simulink model "CRITIS_1_full"  (R2022b)
settings: Solver=VariableStepAuto  StartTime=0.0  StopTime=7  RelTol=1e-3
(part 8 of 13)

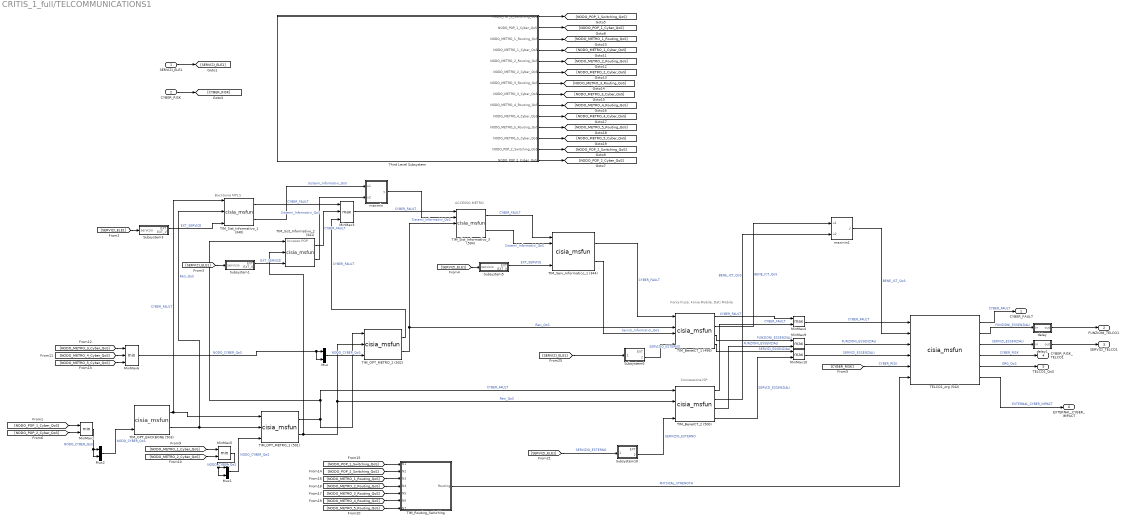
== system CRITIS_1_full/TELCOMMUNICATIONS1 ==
  note: Fonia Fissa, Fonia Mobile, Dati Mobile
  note: Connessione ISP
  note: Backbone MPLS
  note: Accesso POP
  note: ACCESSO METRO
  SERVIZI_ELE1 : Inport
  CYBER_RISK : Inport  Port=2
  MinMax1 : MinMax  Inputs=2
  MinMax10 : MinMax  Function=max  Inputs=2
  MinMax3 : MinMax  Function=max  Inputs=3
  MinMax4 : MinMax  Function=max  Inputs=2
  MinMax5 : MinMax  Inputs=2
  MinMax6 : MinMax  Inputs=3
  MinMax9 : MinMax  Function=max  Inputs=2
  Mux : Mux  Inputs=2
  Mux1 : Mux  Inputs=2
  Mux2 : Mux  Inputs=2
  Subsystem1 : Subsystem  mask{num_serv=1, operation1=All services required, operation2=All providers required, out_service=none, consumed1=[1 0 0 0 0 0 0 0 0 0]}
      mask prompts: num_serv "Providers in input"; operation1 "For each single service provider"; operation2 "Among providers"; out_service "Vectorial output"; consumed1 "Required 1"
      mask TypeOptions num_serv: 1
      mask TypeOptions operation1: All services required | At least one
      mask TypeOptions operation2: All providers required
      mask TypeOptions out_service: none | S1 | S2 | S3 | S4 | S5 | S6 | S7 | S8 | S9 | S10 | F1 | F2 | F3 | F4 | F5 | F6 | F7 | F8 | F9 | F10
  Subsystem10 : Subsystem  mask{num_serv=1, operation1=All services required, operation2=All providers required, out_service=S4, consumed1=[1 0 0 0 0 0 0 0 0 0]}
      mask prompts: num_serv "Providers in input"; operation1 "For each single service provider"; operation2 "Among providers"; out_service "Vectorial output"; consumed1 "Required 1"
      mask TypeOptions num_serv: 1
      mask TypeOptions operation1: All services required | At least one
      mask TypeOptions operation2: All providers required
      mask TypeOptions out_service: none | S1 | S2 | S3 | S4 | S5 | S6 | S7 | S8 | S9 | S10 | F1 | F2 | F3 | F4 | F5 | F6 | F7 | F8 | F9 | F10
  Subsystem3 : Subsystem  mask{num_serv=1, operation1=All services required, operation2=All providers required, out_service=none, consumed1=[1 0 0 0 0 0 0 0 0 0]}
      mask prompts: num_serv "Providers in input"; operation1 "For each single service provider"; operation2 "Among providers"; out_service "Vectorial output"; consumed1 "Required 1"
      mask TypeOptions num_serv: 1
      mask TypeOptions operation1: All services required | At least one
      mask TypeOptions operation2: All providers required
      mask TypeOptions out_service: none | S1 | S2 | S3 | S4 | S5 | S6 | S7 | S8 | S9 | S10 | F1 | F2 | F3 | F4 | F5 | F6 | F7 | F8 | F9 | F10
  Subsystem5 : Subsystem  mask{num_serv=1, operation1=All services required, operation2=All providers required, out_service=none, consumed1=[1 0 0 0 0 0 0 0 0 0]}
      mask prompts: num_serv "Providers in input"; operation1 "For each single service provider"; operation2 "Among providers"; out_service "Vectorial output"; consumed1 "Required 1"
      mask TypeOptions num_serv: 1
      mask TypeOptions operation1: All services required | At least one
      mask TypeOptions operation2: All providers required
      mask TypeOptions out_service: none | S1 | S2 | S3 | S4 | S5 | S6 | S7 | S8 | S9 | S10 | F1 | F2 | F3 | F4 | F5 | F6 | F7 | F8 | F9 | F10
  Subsystem6 : Subsystem  mask{num_serv=1, operation1=All services required, operation2=All providers required, out_service=S1, consumed1=[1 0 0 0 0 0 0 0 0 0]}
      mask prompts: num_serv "Providers in input"; operation1 "For each single service provider"; operation2 "Among providers"; out_service "Vectorial output"; consumed1 "Required 1"
      mask TypeOptions num_serv: 1
      mask TypeOptions operation1: All services required | At least one
      mask TypeOptions operation2: All providers required
      mask TypeOptions out_service: none | S1 | S2 | S3 | S4 | S5 | S6 | S7 | S8 | S9 | S10 | F1 | F2 | F3 | F4 | F5 | F6 | F7 | F8 | F9 | F10
  TELCO1_org (542) : M-S-Function  FunctionName=cisia_msfun  Parameters=Parameter1, Parameter2, Parameter3, resources, Parameter10, codeupdate, step_received, step_computed, dynamic_computed, step_sended, id_entity, id_project, id_type, name_type, color  mask(S-function:msfcn_unit_delay){Parameter1='TELCO1_org', Parameter2=1, Parameter3='Iside', resources=|, Parameter10=off, codeupdate=off, step_received=|, step_computed=, dynamic_computed=, step_sended=|, id_entity=542, id_project=14, id_type=118, name_type=Organization, color=#A2142F}
      mask resources=|
      | *** INPUT RESOURCES ***
      | NUM_INPUTS 6
      | CYBER_FAULT (25)
      | BENE_ICT_QoS (2)
      | FUNZIONI_ESSENZIALI (10)
      | SERVIZI_ESSENZIALI (10)
      | CYBER_RISK (3)
      | PHYSICAL_STRENGTH (1)
      |
      | *** STATE VARIABLES ***
      | NUM_VARIABLES 35
      | Operative_Level(NUMERIC)(1)(1)
      | Dos_attack(NUMERIC)(1)(0)
      | MITM_attack(NUMERIC)(1)(0)
      | Virus_Attack(NUMERIC)(1)(0)
      | Port_Scan_Attack(NUMERIC)(1)(0)
      | Cyber_Fault(NUMERIC_ARRAY)(25)(0  0  0  0  0  0  0  0  0  0  0  0  0  0  0  0  0  0  0  0  0  0  0  0  0)
      | BGP_hijacking(NUMERIC)(1)(0)
      | Mechanical_Fault(NUMERIC)(1)(0)
      | Unauthorized_Access(NUMERIC)(1)(0)
      | Conn_Fault(NUMERIC)(1)(0)
      | BotNet_Attack(NUMERIC)(1)(0)
      | Data_Corruption(NUMERIC)(1)(0)
      | Rouge_Access(NUMERIC)(1)(0)
      | syslog_adm_login(NUMERIC)(1)(0)
      | SW_Change(NUMERIC)(1)(0)
      | Config_Change(NUMERIC)(1)(0)
      | Port_Saturation(NUMERIC)(1)(0)
      | Congestion_Fault(NUMERIC)(1)(0)
      | Physical_Fault(NUMERIC)(1)(0)
      | Route_Poisoning(NUMERIC)(1)(0)
      | Interface_Down(NUMERIC)(1)(0)
      | Port_Isolation(NUMERIC)(1)(0)
      | Unknown_Device(NUMERIC)(1)(0)
      | USB_Device_Insertion(NUMERIC)(1)(0)
      | SW_Fault(NUMERIC)(1)(0)
      | Servizi_Essenziali(NUMERIC_ARRAY)(10)(0  0  0  0  0  0  0  0  0  0)
      | Funzioni_Essenziali(NUMERIC_ARRAY)(10)(0  0  0  0  0  0  0  0  0  0)
      | Internal_Cyber_Risk(NUMERIC)(1)(0)
      | Data_Breach(NUMERIC)(1)(0)
      | availability_fault(NUMERIC)(1)(0)
      | Ransomware(NUMERIC)(1)(0)
      | ExternalCyberFault(NUMERIC_ARRAY)(3)(0  0  0)
      | Op_Level2(NUMERIC_ARRAY)(2)(1  1)
      | Possibility_Value(NUMERIC)(1)(0)
      | Necessity_Value(NUMERIC)(1)(0)
      |
      | *** OUTPUT RESOURCES ***
      | NUM_OUTPUTS 6
      | CYBER_FAULT (25)
      | FUNZIONI_ESSENZIALI (10)
      | SERVIZI_ESSENZIALI (10)
      | CYBER_RISK (3)
      | ORG_QoS (2)
      | EXTERNAL_CYBER_IMPACT (1)
      mask step_received=|
      | cyber_event=zeros(1,25);
      | cyber_event(1)=Dos_attack;
      | cyber_event(2)=MITM_attack;
      | cyber_event(3)=Virus_Attack;
      | cyber_event(4)=Port_Scan_Attack;
      | cyber_event(5)=BGP_hijacking;
      | cyber_event(6)=BotNet_Attack;
      | cyber_event(7)=Data_Corruption;
      | cyber_event(8)=SW_Change;
      | cyber_event(9)=Config_Change;
      | cyber_event(10)=Port_Saturation;
      | cyber_event(11)=Data_Breach;
      | cyber_event(12)=Unauthorized_Access;
      | cyber_event(13)=Unknown_Device;
      | cyber_event(14)=Congestion_Fault;
      | cyber_event(15)=Interface_Down;
      | cyber_event(16)=Port_Isolation;
      | cyber_event(17)=Rouge_Access;
      | cyber_event(18)=Route_Poisoning;
      | cyber_event(19)=SW_Fault;
      | cyber_event(20)=syslog_adm_login;
      | cyber_event(21)=USB_Device_Insertion;
      | cyber_event(22)=Ransomware;
      | cyber_event(23)=0;
      | cyber_event(24)=0;
      | cyber_event(25)=0;
      |
      | Cyber_Fault=max(CYBER_FAULT, transpose(cyber_event));
      |
      |
      | Conn_Fault=max([Dos_attack BGP_hijacking Route_Poisoning Interface_Down Mechanical_Fault] );
      |
      |
      | Servizi_Essenziali=SERVIZI_ESSENZIALI;
      | Funzioni_Essenziali=FUNZIONI_ESSENZIALI;
      |
      | ExternalCyberFault=CYBER_RISK;
      |
      | Operative_Level=min([1-0.5*max(Cyber_Fault) mean(BENE_ICT_QoS) PHYSICAL_STRENGTH]);
      |
      |
      | Physical_Fault=1-PHYSICAL_STRENGTH;
      |
      | % Il primo elemento rappersenta possibility e si combima
      | % con il max in quanto rende conto del caso migliore
      | % (perche OL)
      |
      | Op_Level2(1)=  min([1-0.3*max(Cyber_Fault) BENE_ICT_QoS(1) PHYSICAL_STRENGTH]);
      |
      | % Il secondo elemento rappersenta necessity e si combima
      | % con il min in quanto rende conto del caso peggiore
      | % (perche OL)
      |
      | Op_Level2(2)= min([1-0.6*max(Cyber_Fault) BENE_ICT_QoS(2) PHYSICAL_STRENGTH]);
      |
      | Possibility_Value = Op_Level2(1);
      | Necessity_Value = Op_Level2(2);
      mask step_sended=|
      | SERVIZI_ESSENZIALI=Servizi_Essenziali*(1-Physical_Fault);
      | FUNZIONI_ESSENZIALI=Funzioni_Essenziali*(1-Physical_Fault);
      |
      |
      | ORG_QoS = Op_Level2;
      |
      | % Need to evaluate C-I-A from Cyber_Fault
      | integrity_fault=max([Cyber_Fault(7)  Cyber_Fault(8) Cyber_Fault(22)]);
      |
      | confidentiality_fault=max([Cyber_Fault(2)  Cyber_Fault(3)  Cyber_Fault(6)  Cyber_Fault(9) Cyber_Fault(22)]);
      |
      | availability_fault=max(Cyber_Fault);
      |
      |
      | % C-I-A
      | CYBER_RISK(1)=confidentiality_fault;
      | CYBER_RISK(2)=integrity_fault;
      | CYBER_RISK(3)=availability_fault;
      |
      | % Need to filter the propagable ones
      | CYBER_FAULT = Cyber_Fault;
      |
      |
      | % Need to map from external risks to internal ones
      | EXTERNAL_CYBER_IMPACT=max(ExternalCyberFault);
      mask prompts: Parameter1 "entity name"; Parameter2 "sampling time"; Parameter3 "project"; resources "input resources and state variables"; Parameter10 "Bring state variables to output"; codeupdate "update code from mask"
      mask help: This is a level-2 MATLAB file S-function which demonstrates CISIA entity
      mask DialogControl Container1 Prompt: All parameters
      mask Display: disp('Organization')
  TIM_BeneICT_1 (499) : M-S-Function  FunctionName=cisia_msfun  Parameters=Parameter1, Parameter2, Parameter3, resources, Parameter10, codeupdate, step_received, step_computed, dynamic_computed, step_sended, id_entity, id_project, id_type, name_type, color  mask(S-function:msfcn_unit_delay){Parameter1='TIM_BeneICT_1', Parameter2=1, Parameter3='Iside', resources=|, Parameter10=off, codeupdate=off, step_received=|, step_computed=, dynamic_computed=, step_sended=|, id_entity=499, id_project=14, id_type=108, name_type=BeneICT, color=#64D413}
      mask resources=|
      | *** INPUT RESOURCES ***
      | NUM_INPUTS 6
      | CYBER_FAULT (25)
      | Sistemi_Informativi_QoS (2)
      | Reti_QoS (2)
      | Servizi_Informatici_QoS (2)
      | BENE_ICT_QoS (2)
      | SERVIZIO_ESTERNO (20)
      |
      | *** STATE VARIABLES ***
      | NUM_VARIABLES 34
      | Operative_Level(NUMERIC)(1)(1)
      | Dos_attack(NUMERIC)(1)(0)
      | MITM_attack(NUMERIC)(1)(0)
      | Virus_Attack(NUMERIC)(1)(0)
      | Port_Scan_Attack(NUMERIC)(1)(0)
      | Cyber_Fault(NUMERIC_ARRAY)(25)(0  0  0  0  0  0  0  0  0  0  0  0  0  0  0  0  0  0  0  0  0  0  0  0  0)
      | BGP_hijacking(NUMERIC)(1)(0)
      | Unauthorized_Access(NUMERIC)(1)(0)
      | Consumed_Services(NUMERIC_ARRAY)(10)(0  0  0  0  0  0  0  0  0  0)
      | Service_Fault(NUMERIC)(1)(0)
      | BotNet_Attack(NUMERIC)(1)(0)
      | Data_Corruption(NUMERIC)(1)(0)
      | Rouge_Access(NUMERIC)(1)(0)
      | syslog_adm_login(NUMERIC)(1)(0)
      | SW_Change(NUMERIC)(1)(0)
      | Config_Change(NUMERIC)(1)(0)
      | Port_Saturation(NUMERIC)(1)(0)
      | Congestion_Fault(NUMERIC)(1)(0)
      | Route_Poisoning(NUMERIC)(1)(0)
      | Interface_Down(NUMERIC)(1)(0)
      | Port_Isolation(NUMERIC)(1)(0)
      | Unknown_Device(NUMERIC)(1)(0)
      | USB_Device_Insertion(NUMERIC)(1)(0)
      | SW_Fault(NUMERIC)(1)(0)
      | Servizi_Essenziali(NUMERIC_ARRAY)(10)(1  0  0  0  0  0  0  0  0  0)
      | Funzioni_Essenziali(NUMERIC_ARRAY)(10)(1  0  0  0  0  0  0  0  0  0)
      | Consumed_Functions(NUMERIC_ARRAY)(10)(0  0  0  0  0  0  0  0  0  0)
      | Internal_Cyber_Risk(NUMERIC)(1)(0)
      | Data_Breach(NUMERIC)(1)(0)
      | availability_fault(NUMERIC)(1)(0)
      | Ransomware(NUMERIC)(1)(0)
      | Op_Level2(NUMERIC_ARRAY)(2)(0  0)
      | Possibility_Value(NUMERIC)(1)(0)
      | Necessity_Value(NUMERIC)(1)(0)
      |
      | *** OUTPUT RESOURCES ***
      | NUM_OUTPUTS 4
      | CYBER_FAULT (25)
      | BENE_ICT_QoS (2)
      | FUNZIONI_ESSENZIALI (10)
      | SERVIZI_ESSENZIALI (10)
      mask step_received=|
      | cyber_event=zeros(1,25);
      | cyber_event(1)=Dos_attack;
      | cyber_event(2)=MITM_attack;
      | cyber_event(3)=Virus_Attack;
      | cyber_event(4)=Port_Scan_Attack;
      | cyber_event(5)=BGP_hijacking;
      | cyber_event(6)=BotNet_Attack;
      | cyber_event(7)=Data_Corruption;
      | cyber_event(8)=SW_Change;
      | cyber_event(9)=Config_Change;
      | cyber_event(10)=Port_Saturation;
      | cyber_event(11)=Data_Breach;
      | cyber_event(12)=Unauthorized_Access;
      | cyber_event(13)=Unknown_Device;
      | cyber_event(14)=Congestion_Fault;
      | cyber_event(15)=Interface_Down;
      | cyber_event(16)=Port_Isolation;
      | cyber_event(17)=Rouge_Access;
      | cyber_event(18)=Route_Poisoning;
      | cyber_event(19)=SW_Fault;
      | cyber_event(20)=syslog_adm_login;
      | cyber_event(21)=USB_Device_Insertion;
      | cyber_event(22)=Ransomware;
      | cyber_event(23)=0;
      | cyber_event(24)=0;
      | cyber_event(25)=0;
      |
      | Cyber_Fault=max(CYBER_FAULT, transpose(cyber_event));
      |
      | Consumed_Services=SERVIZIO_ESTERNO(1:10);
      | Consumed_Functions=SERVIZIO_ESTERNO(11:20);
      |
      | Service_Fault=max(abs(Servizi_Essenziali-Consumed_Services));
      |
      | availability_fault=1-min([(1-0.5*max(Cyber_Fault)) min(Reti_QoS) min(Sistemi_Informativi_QoS) min(Servizi_Informatici_QoS) min(BENE_ICT_QoS)]);
      |
      | Operative_Level=min([(1-0.5*max(Cyber_Fault)) mean(Reti_QoS) mean(Sistemi_Informativi_QoS) mean(Servizi_Informatici_QoS) mean(BENE_ICT_QoS) 1-Service_Fault]);
      |
      | % Il primo elemento rappersenta possibility e si combima
      | % con il max in quanto rende conto del caso migliore
      | % (perche OL)
      |
      | BNICT=BENE_ICT_QoS;
      |
      | Op_Level2(1)=  min([1-0.3*max(Cyber_Fault) max([use_elem(Reti_QoS,1) use_elem(Sistemi_Informativi_QoS,1) use_elem(Servizi_Informatici_QoS,1) use_elem(BENE_ICT_QoS,1)]) 1-Service_Fault]);
      |
      | % Il secondo elemento rappresenta necessity e si combima
      | % con il min in quanto rende conto del caso peggiore
      | % (perche OL)
      |
      |
      |
      | Op_Level2(2)= min([1-0.6*max(Cyber_Fault) min([use_elem(Reti_QoS,2) use_elem(Sistemi_Informativi_QoS,2) use_elem(Servizi_Informatici_QoS,2) use_elem(BENE_ICT_QoS,2)]) 1-Service_Fault]);
      |
      | Possibility_Value = Op_Level2(1);
      | Necessity_Value = Op_Level2(2);
      mask step_sended=|
      | CYBER_FAULT=Cyber_Fault;
      |
      | FUNZIONI_ESSENZIALI=(1-availability_fault)*Funzioni_Essenziali.*Consumed_Functions;
      |
      | SERVIZI_ESSENZIALI=(1-availability_fault)*Servizi_Essenziali.*Consumed_Services;
      |
      | BENE_ICT_QoS=Op_Level2;
      mask prompts: Parameter1 "entity name"; Parameter2 "sampling time"; Parameter3 "project"; resources "input resources and state variables"; Parameter10 "Bring state variables to output"; codeupdate "update code from mask"
      mask help: This is a level-2 MATLAB file S-function which demonstrates CISIA entity
      mask DialogControl Container1 Prompt: All parameters
      mask Display: disp('BeneICT');port_label('input',2,'\color{yellow}\spadesuit','texmode','on');port_label('input',5,'\color{yellow}\spadesuit','texmode','on')
  TIM_BeneICT_2 (500) : M-S-Function  FunctionName=cisia_msfun  Parameters=Parameter1, Parameter2, Parameter3, resources, Parameter10, codeupdate, step_received, step_computed, dynamic_computed, step_sended, id_entity, id_project, id_type, name_type, color  mask(S-function:msfcn_unit_delay){Parameter1='TIM_BeneICT_2', Parameter2=1, Parameter3='Iside', resources=|, Parameter10=off, codeupdate=off, step_received=|, step_computed=, dynamic_computed=, step_sended=|, id_entity=500, id_project=14, id_type=108, name_type=BeneICT, color=#64D413}
      mask resources=|
      | *** INPUT RESOURCES ***
      | NUM_INPUTS 6
      | CYBER_FAULT (25)
      | Sistemi_Informativi_QoS (2)
      | Reti_QoS (2)
      | Servizi_Informatici_QoS (2)
      | BENE_ICT_QoS (2)
      | SERVIZIO_ESTERNO (20)
      |
      | *** STATE VARIABLES ***
      | NUM_VARIABLES 34
      | Operative_Level(NUMERIC)(1)(1)
      | Dos_attack(NUMERIC)(1)(0)
      | MITM_attack(NUMERIC)(1)(0)
      | Virus_Attack(NUMERIC)(1)(0)
      | Port_Scan_Attack(NUMERIC)(1)(0)
      | Cyber_Fault(NUMERIC_ARRAY)(25)(0  0  0  0  0  0  0  0  0  0  0  0  0  0  0  0  0  0  0  0  0  0  0  0  0)
      | BGP_hijacking(NUMERIC)(1)(0)
      | Unauthorized_Access(NUMERIC)(1)(0)
      | Consumed_Services(NUMERIC_ARRAY)(10)(0  0  0  0  0  0  0  0  0  0)
      | Service_Fault(NUMERIC)(1)(0)
      | BotNet_Attack(NUMERIC)(1)(0)
      | Data_Corruption(NUMERIC)(1)(0)
      | Rouge_Access(NUMERIC)(1)(0)
      | syslog_adm_login(NUMERIC)(1)(0)
      | SW_Change(NUMERIC)(1)(0)
      | Config_Change(NUMERIC)(1)(0)
      | Port_Saturation(NUMERIC)(1)(0)
      | Congestion_Fault(NUMERIC)(1)(0)
      | Route_Poisoning(NUMERIC)(1)(0)
      | Interface_Down(NUMERIC)(1)(0)
      | Port_Isolation(NUMERIC)(1)(0)
      | Unknown_Device(NUMERIC)(1)(0)
      | USB_Device_Insertion(NUMERIC)(1)(0)
      | SW_Fault(NUMERIC)(1)(0)
      | Servizi_Essenziali(NUMERIC_ARRAY)(10)(0  0  0  1  0  0  0  0  0  0)
      | Funzioni_Essenziali(NUMERIC_ARRAY)(10)(1  0  0  0  0  0  0  0  0  0)
      | Consumed_Functions(NUMERIC_ARRAY)(10)(0  0  0  0  0  0  0  0  0  0)
      | Internal_Cyber_Risk(NUMERIC)(1)(0)
      | Data_Breach(NUMERIC)(1)(0)
      | availability_fault(NUMERIC)(1)(0)
      | Ransomware(NUMERIC)(1)(0)
      | Op_Level2(NUMERIC_ARRAY)(2)(0  0)
      | Possibility_Value(NUMERIC)(1)(0)
      | Necessity_Value(NUMERIC)(1)(0)
      |
      | *** OUTPUT RESOURCES ***
      | NUM_OUTPUTS 4
      | CYBER_FAULT (25)
      | BENE_ICT_QoS (2)
      | FUNZIONI_ESSENZIALI (10)
      | SERVIZI_ESSENZIALI (10)
      mask step_received=|
      | cyber_event=zeros(1,25);
      | cyber_event(1)=Dos_attack;
      | cyber_event(2)=MITM_attack;
      | cyber_event(3)=Virus_Attack;
      | cyber_event(4)=Port_Scan_Attack;
      | cyber_event(5)=BGP_hijacking;
      | cyber_event(6)=BotNet_Attack;
      | cyber_event(7)=Data_Corruption;
      | cyber_event(8)=SW_Change;
      | cyber_event(9)=Config_Change;
      | cyber_event(10)=Port_Saturation;
      | cyber_event(11)=Data_Breach;
      | cyber_event(12)=Unauthorized_Access;
      | cyber_event(13)=Unknown_Device;
      | cyber_event(14)=Congestion_Fault;
      | cyber_event(15)=Interface_Down;
      | cyber_event(16)=Port_Isolation;
      | cyber_event(17)=Rouge_Access;
      | cyber_event(18)=Route_Poisoning;
      | cyber_event(19)=SW_Fault;
      | cyber_event(20)=syslog_adm_login;
      | cyber_event(21)=USB_Device_Insertion;
      | cyber_event(22)=Ransomware;
      | cyber_event(23)=0;
      | cyber_event(24)=0;
      | cyber_event(25)=0;
      |
      | Cyber_Fault=max(CYBER_FAULT, transpose(cyber_event));
      |
      | Consumed_Services=SERVIZIO_ESTERNO(1:10);
      | Consumed_Functions=SERVIZIO_ESTERNO(11:20);
      |
      | Service_Fault=max(abs(Servizi_Essenziali-Consumed_Services));
      |
      | availability_fault=1-min([(1-0.5*max(Cyber_Fault)) min(Reti_QoS) min(Sistemi_Informativi_QoS) min(Servizi_Informatici_QoS) min(BENE_ICT_QoS)]);
      |
      | Operative_Level=min([(1-0.5*max(Cyber_Fault)) mean(Reti_QoS) mean(Sistemi_Informativi_QoS) mean(Servizi_Informatici_QoS) mean(BENE_ICT_QoS) 1-Service_Fault]);
      |
      | % Il primo elemento rappersenta possibility e si combima
      | % con il max in quanto rende conto del caso migliore
      | % (perche OL)
      |
      | BNICT=BENE_ICT_QoS;
      |
      | Op_Level2(1)=  min([1-0.3*max(Cyber_Fault) max([use_elem(Reti_QoS,1) use_elem(Sistemi_Informativi_QoS,1) use_elem(Servizi_Informatici_QoS,1) use_elem(BENE_ICT_QoS,1)]) 1-Service_Fault]);
      |
      | % Il secondo elemento rappresenta necessity e si combima
      | % con il min in quanto rende conto del caso peggiore
      | % (perche OL)
      |
      |
      |
      | Op_Level2(2)= min([1-0.6*max(Cyber_Fault) min([use_elem(Reti_QoS,2) use_elem(Sistemi_Informativi_QoS,2) use_elem(Servizi_Informatici_QoS,2) use_elem(BENE_ICT_QoS,2)]) 1-Service_Fault]);
      |
      | Possibility_Value = Op_Level2(1);
      | Necessity_Value = Op_Level2(2);
      mask step_sended=|
      | CYBER_FAULT=Cyber_Fault;
      |
      | FUNZIONI_ESSENZIALI=(1-availability_fault)*Funzioni_Essenziali.*Consumed_Functions;
      |
      | SERVIZI_ESSENZIALI=(1-availability_fault)*Servizi_Essenziali.*Consumed_Services;
      |
      | BENE_ICT_QoS=Op_Level2;
      mask prompts: Parameter1 "entity name"; Parameter2 "sampling time"; Parameter3 "project"; resources "input resources and state variables"; Parameter10 "Bring state variables to output"; codeupdate "update code from mask"
      mask help: This is a level-2 MATLAB file S-function which demonstrates CISIA entity
      mask DialogControl Container1 Prompt: All parameters
      mask Display: disp('BeneICT');port_label('input',2,'\color{yellow}\spadesuit','texmode','on');port_label('input',4,'\color{yellow}\spadesuit','texmode','on');port_label('input',5,'\color{yellow}\spadesuit','texmode','on')
  TIM_OPT_BACKBONE (503) : M-S-Function  FunctionName=cisia_msfun  Parameters=Parameter1, Parameter2, Parameter3, resources, Parameter10, codeupdate, step_received, step_computed, dynamic_computed, step_sended, id_entity, id_project, id_type, name_type, color  mask(S-function:msfcn_unit_delay){Parameter1='TIM_OPT_BACKBONE', Parameter2=1, Parameter3='Iside', resources=|, Parameter10=off, codeupdate=off, step_received=|, step_computed=, dynamic_computed=, step_sended=|, id_entity=503, id_project=14, id_type=82, name_type=Reti_Sito, color=#45B5ED}
      mask resources=|
      | *** INPUT RESOURCES ***
      | NUM_INPUTS 3
      | CYBER_FAULT (25)
      | Reti_QoS (2)
      | NODO_CYBER_QoS (2)
      |
      | *** STATE VARIABLES ***
      | NUM_VARIABLES 34
      | Operative_Level(NUMERIC)(1)(1)
      | Dos_attack(NUMERIC)(1)(0)
      | MITM_attack(NUMERIC)(1)(0)
      | Virus_Attack(NUMERIC)(1)(0)
      | Port_Scan_Attack(NUMERIC)(1)(0)
      | Cyber_Fault(NUMERIC_ARRAY)(25)(0  0  0  0  0  0  0  0  0  0  0  0  0  0  0  0  0  0  0  0  0  0  0  0  0)
      | BGP_hijacking(NUMERIC)(1)(0)
      | Mechanical_Fault(NUMERIC)(1)(0)
      | Unauthorized_Access(NUMERIC)(1)(0)
      | Conn_Fault(NUMERIC)(1)(0)
      | BotNet_Attack(NUMERIC)(1)(0)
      | Data_Corruption(NUMERIC)(1)(0)
      | Rouge_Access(NUMERIC)(1)(0)
      | syslog_adm_login(NUMERIC)(1)(0)
      | SW_Change(NUMERIC)(1)(0)
      | Config_Change(NUMERIC)(1)(0)
      | Port_Saturation(NUMERIC)(1)(0)
      | Congestion_Fault(NUMERIC)(1)(0)
      | Physical_Fault(NUMERIC)(1)(0)
      | Route2(NUMERIC)(1)(0)
      | Route_Poisoning(NUMERIC)(1)(0)
      | Interface_Down(NUMERIC)(1)(0)
      | Port_Isolation(NUMERIC)(1)(0)
      | Unknown_Device(NUMERIC)(1)(0)
      | USB_Device_Insertion(NUMERIC)(1)(0)
      | Risorsa(NUMERIC)(1)(0)
      | GEO_localization(STRING)(100)()
      | SW_Fault(NUMERIC)(1)(0)
      | Internal_Cyber_Risk(NUMERIC)(1)(0)
      | Data_Breach(NUMERIC)(1)(0)
      | Ransomware(NUMERIC)(1)(0)
      | Op_Level2(NUMERIC_ARRAY)(2)(0  0)
      | Possibility_Value(NUMERIC)(1)(0)
      | Necessity_Value(NUMERIC)(1)(0)
      |
      | *** OUTPUT RESOURCES ***
      | NUM_OUTPUTS 2
      | CYBER_FAULT (25)
      | Reti_QoS (2)
      mask step_received=|
      | cyber_event=zeros(1,25);
      | cyber_event(1)=Dos_attack;
      | cyber_event(2)=MITM_attack;
      | cyber_event(3)=Virus_Attack;
      | cyber_event(4)=Port_Scan_Attack;
      | cyber_event(5)=BGP_hijacking;
      | cyber_event(6)=BotNet_Attack;
      | cyber_event(7)=Data_Corruption;
      | cyber_event(8)=SW_Change;
      | cyber_event(9)=Config_Change;
      | cyber_event(10)=Port_Saturation;
      | cyber_event(11)=Data_Breach;
      | cyber_event(12)=Unauthorized_Access;
      | cyber_event(13)=Unknown_Device;
      | cyber_event(14)=Congestion_Fault;
      | cyber_event(15)=Interface_Down;
      | cyber_event(16)=Port_Isolation;
      | cyber_event(17)=Rouge_Access;
      | cyber_event(18)=Route_Poisoning;
      | cyber_event(19)=SW_Fault;
      | cyber_event(20)=syslog_adm_login;
      | cyber_event(21)=USB_Device_Insertion;
      | cyber_event(22)=Ransomware;
      | cyber_event(23)=0;
      | cyber_event(24)=0;
      | cyber_event(25)=0;
      |
      | Cyber_Fault=max(CYBER_FAULT, transpose(cyber_event));
      |
      | Conn_Fault=max([Dos_attack BGP_hijacking Route_Poisoning Interface_Down Mechanical_Fault] );
      |
      | Operative_Level=min([(1-Conn_Fault) (1-0.5*max(Cyber_Fault))  mean(Reti_QoS)  mean(NODO_CYBER_QoS)]);
      |
      | % Il primo elemento rappersenta possibility e si combima
      | % con il max in quanto rende conto del caso migliore
      | % (perche OL)
      |
      | Op_Level2(1)=  min([1-0.3*max(Cyber_Fault) max([use_elem(Reti_QoS,1) use_elem(NODO_CYBER_QoS,1)]) 1-Conn_Fault]);
      |
      | % Il secondo elemento rappersenta necessity e si combima
      | % con il min in quanto rende conto del caso peggiore
      | % (perche OL)
      |
      | Op_Level2(2)= min([1-0.6*max(Cyber_Fault) min([use_elem(Reti_QoS,2) use_elem(NODO_CYBER_QoS,2)]) 1-Conn_Fault]);
      |
      | Possibility_Value = Op_Level2(1);
      | Necessity_Value = Op_Level2(2);
      mask step_sended=|
      | CYBER_FAULT=Cyber_Fault;
      |
      |
      | Reti_QoS=Op_Level2;
      mask prompts: Parameter1 "entity name"; Parameter2 "sampling time"; Parameter3 "project"; resources "input resources and state variables"; Parameter10 "Bring state variables to output"; codeupdate "update code from mask"
      mask help: This is a level-2 MATLAB file S-function which demonstrates CISIA entity
      mask DialogControl Container1 Prompt: All parameters
      mask Display: disp('Reti_Sito');port_label('input',1,'\color{yellow}\spadesuit','texmode','on');port_label('input',2,'\color{yellow}\spadesuit','texmode','on')
  TIM_OPT_METRO_1 (501) : M-S-Function  FunctionName=cisia_msfun  Parameters=Parameter1, Parameter2, Parameter3, resources, Parameter10, codeupdate, step_received, step_computed, dynamic_computed, step_sended, id_entity, id_project, id_type, name_type, color  mask(S-function:msfcn_unit_delay){Parameter1='TIM_OPT_METRO_1', Parameter2=1, Parameter3='Iside', resources=|, Parameter10=off, codeupdate=off, step_received=|, step_computed=, dynamic_computed=, step_sended=|, id_entity=501, id_project=14, id_type=82, name_type=Reti_Sito, color=#45B5ED}
      mask resources=|
      | *** INPUT RESOURCES ***
      | NUM_INPUTS 3
      | CYBER_FAULT (25)
      | Reti_QoS (2)
      | NODO_CYBER_QoS (2)
      |
      | *** STATE VARIABLES ***
      | NUM_VARIABLES 34
      | Operative_Level(NUMERIC)(1)(1)
      | Dos_attack(NUMERIC)(1)(0)
      | MITM_attack(NUMERIC)(1)(0)
      | Virus_Attack(NUMERIC)(1)(0)
      | Port_Scan_Attack(NUMERIC)(1)(0)
      | Cyber_Fault(NUMERIC_ARRAY)(25)(0  0  0  0  0  0  0  0  0  0  0  0  0  0  0  0  0  0  0  0  0  0  0  0  0)
      | BGP_hijacking(NUMERIC)(1)(0)
      | Mechanical_Fault(NUMERIC)(1)(0)
      | Unauthorized_Access(NUMERIC)(1)(0)
      | Conn_Fault(NUMERIC)(1)(0)
      | BotNet_Attack(NUMERIC)(1)(0)
      | Data_Corruption(NUMERIC)(1)(0)
      | Rouge_Access(NUMERIC)(1)(0)
      | syslog_adm_login(NUMERIC)(1)(0)
      | SW_Change(NUMERIC)(1)(0)
      | Config_Change(NUMERIC)(1)(0)
      | Port_Saturation(NUMERIC)(1)(0)
      | Congestion_Fault(NUMERIC)(1)(0)
      | Physical_Fault(NUMERIC)(1)(0)
      | Route2(NUMERIC)(1)(0)
      | Route_Poisoning(NUMERIC)(1)(0)
      | Interface_Down(NUMERIC)(1)(0)
      | Port_Isolation(NUMERIC)(1)(0)
      | Unknown_Device(NUMERIC)(1)(0)
      | USB_Device_Insertion(NUMERIC)(1)(0)
      | Risorsa(NUMERIC)(1)(0)
      | GEO_localization(STRING)(100)()
      | SW_Fault(NUMERIC)(1)(0)
      | Internal_Cyber_Risk(NUMERIC)(1)(0)
      | Data_Breach(NUMERIC)(1)(0)
      | Ransomware(NUMERIC)(1)(0)
      | Op_Level2(NUMERIC_ARRAY)(2)(0  0)
      | Possibility_Value(NUMERIC)(1)(0)
      | Necessity_Value(NUMERIC)(1)(0)
      |
      | *** OUTPUT RESOURCES ***
      | NUM_OUTPUTS 2
      | CYBER_FAULT (25)
      | Reti_QoS (2)
      mask step_received=|
      | cyber_event=zeros(1,25);
      | cyber_event(1)=Dos_attack;
      | cyber_event(2)=MITM_attack;
      | cyber_event(3)=Virus_Attack;
      | cyber_event(4)=Port_Scan_Attack;
      | cyber_event(5)=BGP_hijacking;
      | cyber_event(6)=BotNet_Attack;
      | cyber_event(7)=Data_Corruption;
      | cyber_event(8)=SW_Change;
      | cyber_event(9)=Config_Change;
      | cyber_event(10)=Port_Saturation;
      | cyber_event(11)=Data_Breach;
      | cyber_event(12)=Unauthorized_Access;
      | cyber_event(13)=Unknown_Device;
      | cyber_event(14)=Congestion_Fault;
      | cyber_event(15)=Interface_Down;
      | cyber_event(16)=Port_Isolation;
      | cyber_event(17)=Rouge_Access;
      | cyber_event(18)=Route_Poisoning;
      | cyber_event(19)=SW_Fault;
      | cyber_event(20)=syslog_adm_login;
      | cyber_event(21)=USB_Device_Insertion;
      | cyber_event(22)=Ransomware;
      | cyber_event(23)=0;
      | cyber_event(24)=0;
      | cyber_event(25)=0;
      |
      | Cyber_Fault=max(CYBER_FAULT, transpose(cyber_event));
      |
      | Conn_Fault=max([Dos_attack BGP_hijacking Route_Poisoning Interface_Down Mechanical_Fault] );
      |
      | Operative_Level=min([(1-Conn_Fault) (1-0.5*max(Cyber_Fault))  mean(Reti_QoS)  mean(NODO_CYBER_QoS)]);
      |
      | % Il primo elemento rappersenta possibility e si combima
      | % con il max in quanto rende conto del caso migliore
      | % (perche OL)
      |
      | Op_Level2(1)=  min([1-0.3*max(Cyber_Fault) max([use_elem(Reti_QoS,1) use_elem(NODO_CYBER_QoS,1)]) 1-Conn_Fault]);
      |
      | % Il secondo elemento rappersenta necessity e si combima
      | % con il min in quanto rende conto del caso peggiore
      | % (perche OL)
      |
      | Op_Level2(2)= min([1-0.6*max(Cyber_Fault) min([use_elem(Reti_QoS,2) use_elem(NODO_CYBER_QoS,2)]) 1-Conn_Fault]);
      |
      | Possibility_Value = Op_Level2(1);
      | Necessity_Value = Op_Level2(2);
      mask step_sended=|
      | CYBER_FAULT=Cyber_Fault;
      |
      |
      | Reti_QoS=Op_Level2;
      mask prompts: Parameter1 "entity name"; Parameter2 "sampling time"; Parameter3 "project"; resources "input resources and state variables"; Parameter10 "Bring state variables to output"; codeupdate "update code from mask"
      mask help: This is a level-2 MATLAB file S-function which demonstrates CISIA entity
      mask DialogControl Container1 Prompt: All parameters
      mask Display: disp('Reti_Sito')
  TIM_OPT_METRO_2 (502) : M-S-Function  FunctionName=cisia_msfun  Parameters=Parameter1, Parameter2, Parameter3, resources, Parameter10, codeupdate, step_received, step_computed, dynamic_computed, step_sended, id_entity, id_project, id_type, name_type, color  mask(S-function:msfcn_unit_delay){Parameter1='TIM_OPT_METRO_2', Parameter2=1, Parameter3='Iside', resources=|, Parameter10=off, codeupdate=off, step_received=|, step_computed=, dynamic_computed=, step_sended=|, id_entity=502, id_project=14, id_type=82, name_type=Reti_Sito, color=#45B5ED}
      mask resources=|
      | *** INPUT RESOURCES ***
      | NUM_INPUTS 3
      | CYBER_FAULT (25)
      | Reti_QoS (2)
      | NODO_CYBER_QoS (2)
      |
      | *** STATE VARIABLES ***
      | NUM_VARIABLES 34
      | Operative_Level(NUMERIC)(1)(1)
      | Dos_attack(NUMERIC)(1)(0)
      | MITM_attack(NUMERIC)(1)(0)
      | Virus_Attack(NUMERIC)(1)(0)
      | Port_Scan_Attack(NUMERIC)(1)(0)
      | Cyber_Fault(NUMERIC_ARRAY)(25)(0  0  0  0  0  0  0  0  0  0  0  0  0  0  0  0  0  0  0  0  0  0  0  0  0)
      | BGP_hijacking(NUMERIC)(1)(0)
      | Mechanical_Fault(NUMERIC)(1)(0)
      | Unauthorized_Access(NUMERIC)(1)(0)
      | Conn_Fault(NUMERIC)(1)(0)
      | BotNet_Attack(NUMERIC)(1)(0)
      | Data_Corruption(NUMERIC)(1)(0)
      | Rouge_Access(NUMERIC)(1)(0)
      | syslog_adm_login(NUMERIC)(1)(0)
      | SW_Change(NUMERIC)(1)(0)
      | Config_Change(NUMERIC)(1)(0)
      | Port_Saturation(NUMERIC)(1)(0)
      | Congestion_Fault(NUMERIC)(1)(0)
      | Physical_Fault(NUMERIC)(1)(0)
      | Route2(NUMERIC)(1)(0)
      | Route_Poisoning(NUMERIC)(1)(0)
      | Interface_Down(NUMERIC)(1)(0)
      | Port_Isolation(NUMERIC)(1)(0)
      | Unknown_Device(NUMERIC)(1)(0)
      | USB_Device_Insertion(NUMERIC)(1)(0)
      | Risorsa(NUMERIC)(1)(0)
      | GEO_localization(STRING)(100)()
      | SW_Fault(NUMERIC)(1)(0)
      | Internal_Cyber_Risk(NUMERIC)(1)(0)
      | Data_Breach(NUMERIC)(1)(0)
      | Ransomware(NUMERIC)(1)(0)
      | Op_Level2(NUMERIC_ARRAY)(2)(0  0)
      | Possibility_Value(NUMERIC)(1)(0)
      | Necessity_Value(NUMERIC)(1)(0)
      |
      | *** OUTPUT RESOURCES ***
      | NUM_OUTPUTS 2
      | CYBER_FAULT (25)
      | Reti_QoS (2)
      mask step_received=|
      | cyber_event=zeros(1,25);
      | cyber_event(1)=Dos_attack;
      | cyber_event(2)=MITM_attack;
      | cyber_event(3)=Virus_Attack;
      | cyber_event(4)=Port_Scan_Attack;
      | cyber_event(5)=BGP_hijacking;
      | cyber_event(6)=BotNet_Attack;
      | cyber_event(7)=Data_Corruption;
      | cyber_event(8)=SW_Change;
      | cyber_event(9)=Config_Change;
      | cyber_event(10)=Port_Saturation;
      | cyber_event(11)=Data_Breach;
      | cyber_event(12)=Unauthorized_Access;
      | cyber_event(13)=Unknown_Device;
      | cyber_event(14)=Congestion_Fault;
      | cyber_event(15)=Interface_Down;
      | cyber_event(16)=Port_Isolation;
      | cyber_event(17)=Rouge_Access;
      | cyber_event(18)=Route_Poisoning;
      | cyber_event(19)=SW_Fault;
      | cyber_event(20)=syslog_adm_login;
      | cyber_event(21)=USB_Device_Insertion;
      | cyber_event(22)=Ransomware;
      | cyber_event(23)=0;
      | cyber_event(24)=0;
      | cyber_event(25)=0;
      |
      | Cyber_Fault=max(CYBER_FAULT, transpose(cyber_event));
      |
      | Conn_Fault=max([Dos_attack BGP_hijacking Route_Poisoning Interface_Down Mechanical_Fault] );
      |
      | Operative_Level=min([(1-Conn_Fault) (1-0.5*max(Cyber_Fault))  mean(Reti_QoS)  mean(NODO_CYBER_QoS)]);
      |
      | % Il primo elemento rappersenta possibility e si combima
      | % con il max in quanto rende conto del caso migliore
      | % (perche OL)
      |
      | Op_Level2(1)=  min([1-0.3*max(Cyber_Fault) max([use_elem(Reti_QoS,1) use_elem(NODO_CYBER_QoS,1)]) 1-Conn_Fault]);
      |
      | % Il secondo elemento rappersenta necessity e si combima
      | % con il min in quanto rende conto del caso peggiore
      | % (perche OL)
      |
      | Op_Level2(2)= min([1-0.6*max(Cyber_Fault) min([use_elem(Reti_QoS,2) use_elem(NODO_CYBER_QoS,2)]) 1-Conn_Fault]);
      |
      | Possibility_Value = Op_Level2(1);
      | Necessity_Value = Op_Level2(2);
      mask step_sended=|
      | CYBER_FAULT=Cyber_Fault;
      |
      |
      | Reti_QoS=Op_Level2;
      mask prompts: Parameter1 "entity name"; Parameter2 "sampling time"; Parameter3 "project"; resources "input resources and state variables"; Parameter10 "Bring state variables to output"; codeupdate "update code from mask"
      mask help: This is a level-2 MATLAB file S-function which demonstrates CISIA entity
      mask DialogControl Container1 Prompt: All parameters
      mask Display: disp('Reti_Sito')
  TIM_Routing_Switching : MATLAB Function  TreatAsAtomicUnit=on
  TIM_Serv_Informatico_1 (344) : M-S-Function  FunctionName=cisia_msfun  Parameters=Parameter1, Parameter2, Parameter3, resources, Parameter10, codeupdate, step_received, step_computed, dynamic_computed, step_sended, id_entity, id_project, id_type, name_type, color  mask(S-function:msfcn_unit_delay){Parameter1='TIM_Serv_Informatico_1', Parameter2=1, Parameter3='Iside', resources=|, Parameter10=off, codeupdate=off, step_received=|, step_computed=, dynamic_computed=, step_sended=|, id_entity=344, id_project=14, id_type=83, name_type=Servizi_Informatici, color=#6FD0E8}
      mask resources=|
      | *** INPUT RESOURCES ***
      | NUM_INPUTS 6
      | CYBER_FAULT (25)
      | Sistemi_Informativi_QoS (2)
      | Reti_QoS (2)
      | Servizi_Informatici_QoS (2)
      | BENE_ICT_QoS (2)
      | EXT_SERVICE (1)
      |
      | *** STATE VARIABLES ***
      | NUM_VARIABLES 31
      | Operative_Level(NUMERIC)(1)(1)
      | Dos_attack(NUMERIC)(1)(0)
      | MITM_attack(NUMERIC)(1)(0)
      | Virus_Attack(NUMERIC)(1)(0)
      | Port_Scan_Attack(NUMERIC)(1)(0)
      | Cyber_Fault(NUMERIC_ARRAY)(25)(0  0  0  0  0  0  0  0  0  0  0  0  0  0  0  0  0  0  0  0  0  0  0  0  0)
      | BGP_hijacking(NUMERIC)(1)(0)
      | Mechanical_Fault(NUMERIC)(1)(0)
      | Unauthorized_Access(NUMERIC)(1)(0)
      | Service_Fault(NUMERIC)(1)(0)
      | BotNet_Attack(NUMERIC)(1)(0)
      | Data_Corruption(NUMERIC)(1)(0)
      | Rouge_Access(NUMERIC)(1)(0)
      | syslog_adm_login(NUMERIC)(1)(0)
      | SW_Change(NUMERIC)(1)(0)
      | Config_Change(NUMERIC)(1)(0)
      | Port_Saturation(NUMERIC)(1)(0)
      | Congestion_Fault(NUMERIC)(1)(0)
      | Route2(NUMERIC)(1)(0)
      | Route_Poisoning(NUMERIC)(1)(0)
      | Interface_Down(NUMERIC)(1)(0)
      | Port_Isolation(NUMERIC)(1)(0)
      | Unknown_Device(NUMERIC)(1)(0)
      | USB_Device_Insertion(NUMERIC)(1)(0)
      | SW_Fault(NUMERIC)(1)(0)
      | Internal_Cyber_Risk(NUMERIC)(1)(0)
      | Data_Breach(NUMERIC)(1)(0)
      | Ransomware(NUMERIC)(1)(0)
      | Op_Level2(NUMERIC_ARRAY)(2)(0  0)
      | Possibility_Value(NUMERIC)(1)(0)
      | Necessity_Value(NUMERIC)(1)(0)
      |
      | *** OUTPUT RESOURCES ***
      | NUM_OUTPUTS 2
      | CYBER_FAULT (25)
      | Servizi_Informatici_QoS (2)
      mask step_received=|
      | cyber_event=zeros(1,25);
      | cyber_event(1)=Dos_attack;
      | cyber_event(2)=MITM_attack;
      | cyber_event(3)=Virus_Attack;
      | cyber_event(4)=Port_Scan_Attack;
      | cyber_event(5)=BGP_hijacking;
      | cyber_event(6)=BotNet_Attack;
      | cyber_event(7)=Data_Corruption;
      | cyber_event(8)=SW_Change;
      | cyber_event(9)=Config_Change;
      | cyber_event(10)=Port_Saturation;
      | cyber_event(11)=Data_Breach;
      | cyber_event(12)=Unauthorized_Access;
      | cyber_event(13)=Unknown_Device;
      | cyber_event(14)=Congestion_Fault;
      | cyber_event(15)=Interface_Down;
      | cyber_event(16)=Port_Isolation;
      | cyber_event(17)=Rouge_Access;
      | cyber_event(18)=Route_Poisoning;
      | cyber_event(19)=SW_Fault;
      | cyber_event(20)=syslog_adm_login;
      | cyber_event(21)=USB_Device_Insertion;
      | cyber_event(22)=Ransomware;
      | cyber_event(23)=0;
      | cyber_event(24)=0;
      | cyber_event(25)=0;
      |
      | Cyber_Fault=max(CYBER_FAULT, transpose(cyber_event));
      |
      | SW_Fault=max([Virus_Attack Data_Corruption SW_Change] );
      |
      | Service_Fault=1-EXT_SERVICE;
      |
      | Operative_Level=min([(1-Service_Fault) (1-SW_Fault) (1- 0.5 * max(Cyber_Fault))  mean(Reti_QoS)  mean(Sistemi_Informativi_QoS) mean(Servizi_Informatici_QoS)  mean(BENE_ICT_QoS)]);
      |
      | % Il primo elemento rappersenta possibility e si combima
      | % con il max in quanto rende conto del caso migliore
      | % (perche OL)
      |
      | Op_Level2(1)=  min([1-0.3*max(Cyber_Fault) max([use_elem(Reti_QoS,1) use_elem(Sistemi_Informativi_QoS,1) use_elem(Servizi_Informatici_QoS,1) use_elem(BENE_ICT_QoS,1)]) 1-Service_Fault (1-SW_Fault)]);
      |
      | % Il secondo elemento rappersenta necessity e si combima
      | % con il min in quanto rende conto del caso peggiore
      | % (perche OL)
      |
      | Op_Level2(2)= min([1-0.6*max(Cyber_Fault) min([use_elem(Reti_QoS,2) use_elem(Sistemi_Informativi_QoS,2) use_elem(Servizi_Informatici_QoS,2) use_elem(BENE_ICT_QoS,2)]) 1-Service_Fault 1-SW_Fault]);
      |
      | Possibility_Value = Op_Level2(1);
      | Necessity_Value = Op_Level2(2);
      mask step_sended=|
      | CYBER_FAULT=Cyber_Fault;
      |
      | Servizi_Informatici_QoS=Op_Level2;
      mask prompts: Parameter1 "entity name"; Parameter2 "sampling time"; Parameter3 "project"; resources "input resources and state variables"; Parameter10 "Bring state variables to output"; codeupdate "update code from mask"
      mask help: This is a level-2 MATLAB file S-function which demonstrates CISIA entity
      mask DialogControl Container1 Prompt: All parameters
      mask Display: disp('Servizi_Informatici');port_label('input',3,'\color{yellow}\spadesuit','texmode','on');port_label('input',4,'\color{yellow}\spadesuit','texmode','on');port_label('input',5,'\color{yellow}\spadesuit','texmode','on')
  TIM_Sist_Informativo_1 (340) : M-S-Function  FunctionName=cisia_msfun  Parameters=Parameter1, Parameter2, Parameter3, resources, Parameter10, codeupdate, step_received, step_computed, dynamic_computed, step_sended, id_entity, id_project, id_type, name_type, color  mask(S-function:msfcn_unit_delay){Parameter1='TIM_Sist_Informativo_1', Parameter2=1, Parameter3='Iside', resources=|, Parameter10=off, codeupdate=off, step_received=|, step_computed=, dynamic_computed=, step_sended=|, id_entity=340, id_project=14, id_type=81, name_type=Sistemi_Informativi, color=#59F2F7}
      mask resources=|
      | *** INPUT RESOURCES ***
      | NUM_INPUTS 5
      | CYBER_FAULT (25)
      | Sistemi_Informativi_QoS (2)
      | Reti_QoS (2)
      | Servizi_Informatici_QoS (2)
      | EXT_SERVICE (1)
      |
      | *** STATE VARIABLES ***
      | NUM_VARIABLES 33
      | Operative_Level(NUMERIC)(1)(1)
      | Dos_attack(NUMERIC)(1)(0)
      | MITM_attack(NUMERIC)(1)(0)
      | Virus_Attack(NUMERIC)(1)(0)
      | Port_Scan_Attack(NUMERIC)(1)(0)
      | Cyber_Fault(NUMERIC_ARRAY)(25)(0  0  0  0  0  0  0  0  0  0  0  0  0  0  0  0  0  0  0  0  0  0  0  0  0)
      | BGP_hijacking(NUMERIC)(1)(0)
      | Mechanical_Fault(NUMERIC)(1)(0)
      | Power_Fault(NUMERIC)(1)(0)
      | Unauthorized_Access(NUMERIC)(1)(0)
      | Consumed_Services(NUMERIC_ARRAY)(10)(0  0  0  0  0  0  0  0  0  0)
      | Service_Fault(NUMERIC)(1)(0)
      | BotNet_Attack(NUMERIC)(1)(0)
      | Data_Corruption(NUMERIC)(1)(0)
      | Rouge_Access(NUMERIC)(1)(0)
      | syslog_adm_login(NUMERIC)(1)(0)
      | SW_Change(NUMERIC)(1)(0)
      | Config_Change(NUMERIC)(1)(0)
      | Port_Saturation(NUMERIC)(1)(0)
      | Congestion_Fault(NUMERIC)(1)(0)
      | Route_Poisoning(NUMERIC)(1)(0)
      | Interface_Down(NUMERIC)(1)(0)
      | Port_Isolation(NUMERIC)(1)(0)
      | Unknown_Device(NUMERIC)(1)(0)
      | USB_Device_Insertion(NUMERIC)(1)(0)
      | Computational_Fault(NUMERIC)(1)(0)
      | SW_Fault(NUMERIC)(1)(0)
      | Internal_Cyber_Risk(NUMERIC)(1)(0)
      | Data_Breach(NUMERIC)(1)(0)
      | Ransomware(NUMERIC)(1)(0)
      | Op_Level2(NUMERIC_ARRAY)(2)(0  0)
      | Possibility_Value(NUMERIC)(1)(0)
      | Necessity_Value(NUMERIC)(1)(0)
      |
      | *** OUTPUT RESOURCES ***
      | NUM_OUTPUTS 2
      | CYBER_FAULT (25)
      | Sistemi_Informativi_QoS (2)
      mask step_received=|
      | cyber_event=zeros(1,25);
      | cyber_event(1)=Dos_attack;
      | cyber_event(2)=MITM_attack;
      | cyber_event(3)=Virus_Attack;
      | cyber_event(4)=Port_Scan_Attack;
      | cyber_event(5)=BGP_hijacking;
      | cyber_event(6)=BotNet_Attack;
      | cyber_event(7)=Data_Corruption;
      | cyber_event(8)=SW_Change;
      | cyber_event(9)=Config_Change;
      | cyber_event(10)=Port_Saturation;
      | cyber_event(11)=Data_Breach;
      | cyber_event(12)=Unauthorized_Access;
      | cyber_event(13)=Unknown_Device;
      | cyber_event(14)=Congestion_Fault;
      | cyber_event(15)=Interface_Down;
      | cyber_event(16)=Port_Isolation;
      | cyber_event(17)=Rouge_Access;
      | cyber_event(18)=Route_Poisoning;
      | cyber_event(19)=SW_Fault;
      | cyber_event(20)=syslog_adm_login;
      | cyber_event(21)=USB_Device_Insertion;
      | cyber_event(22)=Ransomware;
      | cyber_event(23)=0;
      | cyber_event(24)=0;
      | cyber_event(25)=0;
      |
      | Cyber_Fault=max(CYBER_FAULT, transpose(cyber_event));
      |
      | Computational_Fault=max([Dos_attack Virus_Attack BotNet_Attack Config_Change Mechanical_Fault] );
      |
      | Service_Fault=1-EXT_SERVICE;
      |
      | Operative_Level=min([(1-Service_Fault) (1-Computational_Fault) (1-0.5*max(Cyber_Fault))  mean(Reti_QoS)  mean(Sistemi_Informativi_QoS)  mean(Servizi_Informatici_QoS)]);
      |
      | % Il primo elemento rappersenta possibility e si combima
      | % con il max in quanto rende conto del caso migliore
      | % (perche OL)
      |
      | Op_Level2(1)=  min([1-0.3*max(Cyber_Fault) max([use_elem(Reti_QoS,1) use_elem(Sistemi_Informativi_QoS,1) use_elem(Servizi_Informatici_QoS,1)]) 1-Service_Fault (1-Computational_Fault)]);
      |
      | % Il secondo elemento rappersenta necessity e si combima
      | % con il min in quanto rende conto del caso peggiore
      | % (perche OL)
      |
      | Op_Level2(2)= min([1-0.6*max(Cyber_Fault) min([use_elem(Reti_QoS,2) use_elem(Sistemi_Informativi_QoS,2) use_elem(Servizi_Informatici_QoS,2)]) 1-Service_Fault 1-Computational_Fault]);
      |
      | Possibility_Value = Op_Level2(1);
      | Necessity_Value = Op_Level2(2);
      mask step_sended=|
      | CYBER_FAULT=Cyber_Fault;
      |
      | Sistemi_Informativi_QoS=Op_Level2;
      mask prompts: Parameter1 "entity name"; Parameter2 "sampling time"; Parameter3 "project"; resources "input resources and state variables"; Parameter10 "Bring state variables to output"; codeupdate "update code from mask"
      mask help: This is a level-2 MATLAB file S-function which demonstrates CISIA entity
      mask DialogControl Container1 Prompt: All parameters
      mask Display: disp('Sistemi_Informativi');port_label('input',2,'\color{yellow}\spadesuit','texmode','on');port_label('input',4,'\color{yellow}\spadesuit','texmode','on')
  TIM_Sist_Informativo_2 (341) : M-S-Function  FunctionName=cisia_msfun  Parameters=Parameter1, Parameter2, Parameter3, resources, Parameter10, codeupdate, step_received, step_computed, dynamic_computed, step_sended, id_entity, id_project, id_type, name_type, color  mask(S-function:msfcn_unit_delay){Parameter1='TIM_Sist_Informativo_2', Parameter2=1, Parameter3='Iside', resources=|, Parameter10=off, codeupdate=off, step_received=|, step_computed=, dynamic_computed=, step_sended=|, id_entity=341, id_project=14, id_type=81, name_type=Sistemi_Informativi, color=#59F2F7}
      mask resources=|
      | *** INPUT RESOURCES ***
      | NUM_INPUTS 5
      | CYBER_FAULT (25)
      | Sistemi_Informativi_QoS (2)
      | Reti_QoS (2)
      | Servizi_Informatici_QoS (2)
      | EXT_SERVICE (1)
      |
      | *** STATE VARIABLES ***
      | NUM_VARIABLES 33
      | Operative_Level(NUMERIC)(1)(1)
      | Dos_attack(NUMERIC)(1)(0)
      | MITM_attack(NUMERIC)(1)(0)
      | Virus_Attack(NUMERIC)(1)(0)
      | Port_Scan_Attack(NUMERIC)(1)(0)
      | Cyber_Fault(NUMERIC_ARRAY)(25)(0  0  0  0  0  0  0  0  0  0  0  0  0  0  0  0  0  0  0  0  0  0  0  0  0)
      | BGP_hijacking(NUMERIC)(1)(0)
      | Mechanical_Fault(NUMERIC)(1)(0)
      | Power_Fault(NUMERIC)(1)(0)
      | Unauthorized_Access(NUMERIC)(1)(0)
      | Consumed_Services(NUMERIC_ARRAY)(10)(0  0  0  0  0  0  0  0  0  0)
      | Service_Fault(NUMERIC)(1)(0)
      | BotNet_Attack(NUMERIC)(1)(0)
      | Data_Corruption(NUMERIC)(1)(0)
      | Rouge_Access(NUMERIC)(1)(0)
      | syslog_adm_login(NUMERIC)(1)(0)
      | SW_Change(NUMERIC)(1)(0)
      | Config_Change(NUMERIC)(1)(0)
      | Port_Saturation(NUMERIC)(1)(0)
      | Congestion_Fault(NUMERIC)(1)(0)
      | Route_Poisoning(NUMERIC)(1)(0)
      | Interface_Down(NUMERIC)(1)(0)
      | Port_Isolation(NUMERIC)(1)(0)
      | Unknown_Device(NUMERIC)(1)(0)
      | USB_Device_Insertion(NUMERIC)(1)(0)
      | Computational_Fault(NUMERIC)(1)(0)
      | SW_Fault(NUMERIC)(1)(0)
      | Internal_Cyber_Risk(NUMERIC)(1)(0)
      | Data_Breach(NUMERIC)(1)(0)
      | Ransomware(NUMERIC)(1)(0)
      | Op_Level2(NUMERIC_ARRAY)(2)(0  0)
      | Possibility_Value(NUMERIC)(1)(0)
      | Necessity_Value(NUMERIC)(1)(0)
      |
      | *** OUTPUT RESOURCES ***
      | NUM_OUTPUTS 2
      | CYBER_FAULT (25)
      | Sistemi_Informativi_QoS (2)
      mask step_received=|
      | cyber_event=zeros(1,25);
      | cyber_event(1)=Dos_attack;
      | cyber_event(2)=MITM_attack;
      | cyber_event(3)=Virus_Attack;
      | cyber_event(4)=Port_Scan_Attack;
      | cyber_event(5)=BGP_hijacking;
      | cyber_event(6)=BotNet_Attack;
      | cyber_event(7)=Data_Corruption;
      | cyber_event(8)=SW_Change;
      | cyber_event(9)=Config_Change;
      | cyber_event(10)=Port_Saturation;
      | cyber_event(11)=Data_Breach;
      | cyber_event(12)=Unauthorized_Access;
      | cyber_event(13)=Unknown_Device;
      | cyber_event(14)=Congestion_Fault;
      | cyber_event(15)=Interface_Down;
      | cyber_event(16)=Port_Isolation;
      | cyber_event(17)=Rouge_Access;
      | cyber_event(18)=Route_Poisoning;
      | cyber_event(19)=SW_Fault;
      | cyber_event(20)=syslog_adm_login;
      | cyber_event(21)=USB_Device_Insertion;
      | cyber_event(22)=Ransomware;
      | cyber_event(23)=0;
      | cyber_event(24)=0;
      | cyber_event(25)=0;
      |
      | Cyber_Fault=max(CYBER_FAULT, transpose(cyber_event));
      |
      | Computational_Fault=max([Dos_attack Virus_Attack BotNet_Attack Config_Change Mechanical_Fault] );
      |
      | Service_Fault=1-EXT_SERVICE;
      |
      | Operative_Level=min([(1-Service_Fault) (1-Computational_Fault) (1-0.5*max(Cyber_Fault))  mean(Reti_QoS)  mean(Sistemi_Informativi_QoS)  mean(Servizi_Informatici_QoS)]);
      |
      | % Il primo elemento rappersenta possibility e si combima
      | % con il max in quanto rende conto del caso migliore
      | % (perche OL)
      |
      | Op_Level2(1)=  min([1-0.3*max(Cyber_Fault) max([use_elem(Reti_QoS,1) use_elem(Sistemi_Informativi_QoS,1) use_elem(Servizi_Informatici_QoS,1)]) 1-Service_Fault (1-Computational_Fault)]);
      |
      | % Il secondo elemento rappersenta necessity e si combima
      | % con il min in quanto rende conto del caso peggiore
      | % (perche OL)
      |
      | Op_Level2(2)= min([1-0.6*max(Cyber_Fault) min([use_elem(Reti_QoS,2) use_elem(Sistemi_Informativi_QoS,2) use_elem(Servizi_Informatici_QoS,2)]) 1-Service_Fault 1-Computational_Fault]);
      |
      | Possibility_Value = Op_Level2(1);
      | Necessity_Value = Op_Level2(2);
      mask step_sended=|
      | CYBER_FAULT=Cyber_Fault;
      |
      | Sistemi_Informativi_QoS=Op_Level2;
      mask prompts: Parameter1 "entity name"; Parameter2 "sampling time"; Parameter3 "project"; resources "input resources and state variables"; Parameter10 "Bring state variables to output"; codeupdate "update code from mask"
      mask help: This is a level-2 MATLAB file S-function which demonstrates CISIA entity
      mask DialogControl Container1 Prompt: All parameters
      mask Display: disp('Sistemi_Informativi');port_label('input',2,'\color{yellow}\spadesuit','texmode','on');port_label('input',4,'\color{yellow}\spadesuit','texmode','on')
  TIM_Sist_Informativo_3 (504) : M-S-Function  FunctionName=cisia_msfun  Parameters=Parameter1, Parameter2, Parameter3, resources, Parameter10, codeupdate, step_received, step_computed, dynamic_computed, step_sended, id_entity, id_project, id_type, name_type, color  mask(S-function:msfcn_unit_delay){Parameter1='TIM_Sist_Informativo_3', Parameter2=1, Parameter3='Iside', resources=|, Parameter10=off, codeupdate=off, step_received=|, step_computed=, dynamic_computed=, step_sended=|, id_entity=504, id_project=14, id_type=81, name_type=Sistemi_Informativi, color=#59F2F7}
      mask resources=|
      | *** INPUT RESOURCES ***
      | NUM_INPUTS 5
      | CYBER_FAULT (25)
      | Sistemi_Informativi_QoS (2)
      | Reti_QoS (2)
      | Servizi_Informatici_QoS (2)
      | EXT_SERVICE (1)
      |
      | *** STATE VARIABLES ***
      | NUM_VARIABLES 33
      | Operative_Level(NUMERIC)(1)(1)
      | Dos_attack(NUMERIC)(1)(0)
      | MITM_attack(NUMERIC)(1)(0)
      | Virus_Attack(NUMERIC)(1)(0)
      | Port_Scan_Attack(NUMERIC)(1)(0)
      | Cyber_Fault(NUMERIC_ARRAY)(25)(0  0  0  0  0  0  0  0  0  0  0  0  0  0  0  0  0  0  0  0  0  0  0  0  0)
      | BGP_hijacking(NUMERIC)(1)(0)
      | Mechanical_Fault(NUMERIC)(1)(0)
      | Power_Fault(NUMERIC)(1)(0)
      | Unauthorized_Access(NUMERIC)(1)(0)
      | Consumed_Services(NUMERIC_ARRAY)(10)(0  0  0  0  0  0  0  0  0  0)
      | Service_Fault(NUMERIC)(1)(0)
      | BotNet_Attack(NUMERIC)(1)(0)
      | Data_Corruption(NUMERIC)(1)(0)
      | Rouge_Access(NUMERIC)(1)(0)
      | syslog_adm_login(NUMERIC)(1)(0)
      | SW_Change(NUMERIC)(1)(0)
      | Config_Change(NUMERIC)(1)(0)
      | Port_Saturation(NUMERIC)(1)(0)
      | Congestion_Fault(NUMERIC)(1)(0)
      | Route_Poisoning(NUMERIC)(1)(0)
      | Interface_Down(NUMERIC)(1)(0)
      | Port_Isolation(NUMERIC)(1)(0)
      | Unknown_Device(NUMERIC)(1)(0)
      | USB_Device_Insertion(NUMERIC)(1)(0)
      | Computational_Fault(NUMERIC)(1)(0)
      | SW_Fault(NUMERIC)(1)(0)
      | Internal_Cyber_Risk(NUMERIC)(1)(0)
      | Data_Breach(NUMERIC)(1)(0)
      | Ransomware(NUMERIC)(1)(0)
      | Op_Level2(NUMERIC_ARRAY)(2)(0  0)
      | Possibility_Value(NUMERIC)(1)(0)
      | Necessity_Value(NUMERIC)(1)(0)
      |
      | *** OUTPUT RESOURCES ***
      | NUM_OUTPUTS 2
      | CYBER_FAULT (25)
      | Sistemi_Informativi_QoS (2)
      mask step_received=|
      | cyber_event=zeros(1,25);
      | cyber_event(1)=Dos_attack;
      | cyber_event(2)=MITM_attack;
      | cyber_event(3)=Virus_Attack;
      | cyber_event(4)=Port_Scan_Attack;
      | cyber_event(5)=BGP_hijacking;
      | cyber_event(6)=BotNet_Attack;
      | cyber_event(7)=Data_Corruption;
      | cyber_event(8)=SW_Change;
      | cyber_event(9)=Config_Change;
      | cyber_event(10)=Port_Saturation;
      | cyber_event(11)=Data_Breach;
      | cyber_event(12)=Unauthorized_Access;
      | cyber_event(13)=Unknown_Device;
      | cyber_event(14)=Congestion_Fault;
      | cyber_event(15)=Interface_Down;
      | cyber_event(16)=Port_Isolation;
      | cyber_event(17)=Rouge_Access;
      | cyber_event(18)=Route_Poisoning;
      | cyber_event(19)=SW_Fault;
      | cyber_event(20)=syslog_adm_login;
      | cyber_event(21)=USB_Device_Insertion;
      | cyber_event(22)=Ransomware;
      | cyber_event(23)=0;
      | cyber_event(24)=0;
      | cyber_event(25)=0;
      |
      | Cyber_Fault=max(CYBER_FAULT, transpose(cyber_event));
      |
      | Computational_Fault=max([Dos_attack Virus_Attack BotNet_Attack Config_Change Mechanical_Fault] );
      |
      | Service_Fault=1-EXT_SERVICE;
      |
      | Operative_Level=min([(1-Service_Fault) (1-Computational_Fault) (1-0.5*max(Cyber_Fault))  mean(Reti_QoS)  mean(Sistemi_Informativi_QoS)  mean(Servizi_Informatici_QoS)]);
      |
      | % Il primo elemento rappersenta possibility e si combima
      | % con il max in quanto rende conto del caso migliore
      | % (perche OL)
      |
      | Op_Level2(1)=  min([1-0.3*max(Cyber_Fault) max([use_elem(Reti_QoS,1) use_elem(Sistemi_Informativi_QoS,1) use_elem(Servizi_Informatici_QoS,1)]) 1-Service_Fault (1-Computational_Fault)]);
      |
      | % Il secondo elemento rappersenta necessity e si combima
      | % con il min in quanto rende conto del caso peggiore
      | % (perche OL)
      |
      | Op_Level2(2)= min([1-0.6*max(Cyber_Fault) min([use_elem(Reti_QoS,2) use_elem(Sistemi_Informativi_QoS,2) use_elem(Servizi_Informatici_QoS,2)]) 1-Service_Fault 1-Computational_Fault]);
      |
      | Possibility_Value = Op_Level2(1);
      | Necessity_Value = Op_Level2(2);
      mask step_sended=|
      | CYBER_FAULT=Cyber_Fault;
      |
      | Sistemi_Informativi_QoS=Op_Level2;
      mask prompts: Parameter1 "entity name"; Parameter2 "sampling time"; Parameter3 "project"; resources "input resources and state variables"; Parameter10 "Bring state variables to output"; codeupdate "update code from mask"
      mask help: This is a level-2 MATLAB file S-function which demonstrates CISIA entity
      mask DialogControl Container1 Prompt: All parameters
      mask Display: disp('Sistemi_Informativi');port_label('input',4,'\color{yellow}\spadesuit','texmode','on');port_label('input',5,'\color{yellow}\spadesuit','texmode','on')
  Third Level Subsystem : Subsystem
      mask Display: image('PNG/ReteTLC.png'); % Use "Edit Image" on toolstrip to change.
  delay : Subsystem  mask{delay=0.9, output=ones(1,10)}
  delay1 : Subsystem  mask{delay=0.9, output=ones(1,10)}
  maxmin : MATLAB Function  TreatAsAtomicUnit=on
  maxmin1 : MATLAB Function  TreatAsAtomicUnit=on
  CYBER_FAULT : Outport
  FUNZIONI_TELCO1 : Outport  Port=2
  SERVIZI_TELCO1 : Outport  Port=3
  CYBER_RISK_TELCO1 : Outport  Port=4
  TELCO1_QoS : Outport  Port=5
  EXTERNAL_CYBER_IMPACT : Outport  Port=6
  wires:
  TELCO1_org (542)/1 -> CYBER_FAULT/1  "CYBER_FAULT"
  TELCO1_org (542)/3 -> delay1/1(in)  "SERVIZI_ESSENZIALI"
  TELCO1_org (542)/4 -> CYBER_RISK_TELCO1/1  "CYBER_RISK"
  TIM_BeneICT_2 (500)/1 -> MinMax4/2  "CYBER_FAULT"
  SERVIZI_ELE1/1 -> [SERVIZI_ELE1]
  MinMax4/1 -> TELCO1_org (542)/1  "CYBER_FAULT"
  MinMax10/1 -> TELCO1_org (542)/4  "SERVIZI_ESSENZIALI"
  TIM_Routing_Switching/1(Routing) -> TELCO1_org (542)/6  "PHYSICAL_STRENGTH"
  TIM_OPT_METRO_1 (501)/1 -> TIM_OPT_METRO_2 (502)/1, TIM_BeneICT_2 (500)/1, TIM_Sist_Informativo_2 (341)/1  "CYBER_FAULT"
  TIM_Sist_Informativo_3 (504)/1 -> TIM_Serv_Informatico_1 (344)/1  "CYBER_FAULT"
  TIM_BeneICT_1 (499)/1 -> MinMax4/1  "CYBER_FAULT"
  Mux2/1 -> TIM_OPT_BACKBONE (503)/3  "NODO_CYBER_QoS"
  Third Level Subsystem/1(NODO_POP_1_Switching_QoS) -> [NODO_POP_1_Switching_QoS]
  Third Level Subsystem/2(NODO_POP_1_Cyber_QoS) -> [NODO_POP_1_Cyber_QoS]
  Third Level Subsystem/14(NODO_POP_2_Cyber_QoS) -> [NODO_POP_2_Cyber_QoS]
  Third Level Subsystem/13(NODO_POP_2_Switching_QoS) -> [NODO_POP_2_Switching_QoS]
  [NODO_POP_1_Cyber_QoS] -> MinMax1/1
  [NODO_POP_2_Cyber_QoS] -> MinMax1/2
  [NODO_METRO_2_Cyber_QoS] -> MinMax5/2
  Mux1/1 -> TIM_OPT_METRO_1 (501)/3  "NODO_CYBER_QoS"
  [NODO_METRO_1_Cyber_QoS] -> MinMax5/1
  Third Level Subsystem/3(NODO_METRO_1_Routing_QoS) -> [NODO_METRO_1_Routing_QoS]
  Third Level Subsystem/4(NODO_METRO_1_Cyber_QoS) -> [NODO_METRO_1_Cyber_QoS]
  Third Level Subsystem/6(NODO_METRO_2_Cyber_QoS) -> [NODO_METRO_2_Cyber_QoS]
  Third Level Subsystem/5(NODO_METRO_2_Routing_QoS) -> [NODO_METRO_2_Routing_QoS]
  Mux/1 -> TIM_OPT_METRO_2 (502)/3  "NODO_CYBER_QoS"
  [NODO_METRO_3_Cyber_QoS] -> MinMax6/1
  [NODO_METRO_4_Cyber_QoS] -> MinMax6/2
  [NODO_METRO_5_Cyber_QoS] -> MinMax6/3
  Third Level Subsystem/8(NODO_METRO_3_Cyber_QoS) -> [NODO_METRO_3_Cyber_QoS]
  Third Level Subsystem/10(NODO_METRO_4_Cyber_QoS) -> [NODO_METRO_4_Cyber_QoS]
  Third Level Subsystem/12(NODO_METRO_5_Cyber_QoS) -> [NODO_METRO_5_Cyber_QoS]
  Third Level Subsystem/11(NODO_METRO_5_Routing_QoS) -> [NODO_METRO_5_Routing_QoS]
  Third Level Subsystem/9(NODO_METRO_4_Routing_QoS) -> [NODO_METRO_4_Routing_QoS]
  Third Level Subsystem/7(NODO_METRO_3_Routing_QoS) -> [NODO_METRO_3_Routing_QoS]
  [NODO_POP_1_Switching_QoS] -> TIM_Routing_Switching/1(N1)
  [NODO_POP_2_Switching_QoS] -> TIM_Routing_Switching/2(N2)
  [NODO_METRO_1_Routing_QoS] -> TIM_Routing_Switching/3(N3)
  [NODO_METRO_2_Routing_QoS] -> TIM_Routing_Switching/4(N4)
  [NODO_METRO_3_Routing_QoS] -> TIM_Routing_Switching/5(N5)
  [NODO_METRO_5_Routing_QoS] -> TIM_Routing_Switching/7(N7)
  [NODO_METRO_4_Routing_QoS] -> TIM_Routing_Switching/6(N6)
  TIM_OPT_BACKBONE (503)/1 -> TIM_OPT_METRO_1 (501)/1, TIM_Sist_Informativo_1 (340)/1  "CYBER_FAULT"
  TELCO1_org (542)/5 -> TELCO1_QoS/1  "ORG_QoS"
  TIM_OPT_BACKBONE (503)/2 -> TIM_Sist_Informativo_1 (340)/3, TIM_OPT_METRO_1 (501)/2  "Reti_QoS"
  TIM_OPT_METRO_1 (501)/2 -> TIM_BeneICT_2 (500)/3, TIM_OPT_METRO_2 (502)/2, TIM_Sist_Informativo_2 (341)/3  "Reti_QoS"
  MinMax3/1 -> TIM_Sist_Informativo_3 (504)/1  "CYBER_FAULT"
  TIM_Sist_Informativo_1 (340)/2 -> maxmin/1(u1)  "Sistemi_Informativi_QoS"
  TIM_Sist_Informativo_2 (341)/2 -> maxmin/2(u2)  "Sistemi_Informativi_QoS"
  TIM_OPT_METRO_2 (502)/2 -> TIM_BeneICT_1 (499)/3, TIM_Sist_Informativo_3 (504)/3  "Reti_QoS"
  TIM_OPT_METRO_2 (502)/1 -> MinMax3/3  "CYBER_FAULT"
  TIM_Sist_Informativo_2 (341)/1 -> MinMax3/2  "CYBER_FAULT"
  TIM_Sist_Informativo_1 (340)/1 -> MinMax3/1  "CYBER_FAULT"
  maxmin/1(y) -> TIM_Sist_Informativo_3 (504)/2  "Sistemi_Informativi_QoS"
  TIM_Serv_Informatico_1 (344)/1 -> TIM_BeneICT_1 (499)/1  "CYBER_FAULT"
  TIM_Sist_Informativo_3 (504)/2 -> TIM_Serv_Informatico_1 (344)/2  "Sistemi_Informativi_QoS"
  TIM_BeneICT_1 (499)/4 -> MinMax10/1  "SERVIZI_ESSENZIALI"
  TIM_BeneICT_2 (500)/4 -> MinMax10/2  "SERVIZI_ESSENZIALI"
  TIM_BeneICT_1 (499)/3 -> MinMax9/1  "FUNZIONI_ESSENZIALI"
  TIM_BeneICT_2 (500)/3 -> MinMax9/2  "FUNZIONI_ESSENZIALI"
  maxmin1/1(y) -> TELCO1_org (542)/2  "BENE_ICT_QoS"
  TIM_BeneICT_1 (499)/2 -> maxmin1/1(u1)  "BENE_ICT_QoS"
  TIM_BeneICT_2 (500)/2 -> maxmin1/2(u2)  "BENE_ICT_QoS"
  TELCO1_org (542)/6 -> EXTERNAL_CYBER_IMPACT/1  "EXTERNAL_CYBER_IMPACT"
  MinMax9/1 -> TELCO1_org (542)/3  "FUNZIONI_ESSENZIALI"
  Subsystem6/2(EXT_V) -> TIM_BeneICT_1 (499)/6  "SERVIZIO_ESTERNO"
  [SERVIZI_ELE1] -> Subsystem6/1(servizio)
  Subsystem10/2(EXT_V) -> TIM_BeneICT_2 (500)/6  "SERVIZIO_ESTERNO"
  [SERVIZI_ELE1] -> Subsystem10/1(servizio)  "SERVIZIO_ESTERNO"
  [SERVIZI_ELE1] -> Subsystem3/1(servizio)
  TIM_Serv_Informatico_1 (344)/2 -> TIM_BeneICT_1 (499)/4  "Servizi_Informatici_QoS"
  TELCO1_org (542)/2 -> delay/1(in)  "FUNZIONI_ESSENZIALI"
  delay/1(out) -> FUNZIONI_TELCO1/1
  [SERVIZI_ELE1] -> Subsystem1/1(servizio)
  Subsystem1/1(EXT) -> TIM_Sist_Informativo_2 (341)/5  "EXT_SERVICE"
  Subsystem3/1(EXT) -> TIM_Sist_Informativo_1 (340)/5  "EXT_SERVICE"
  Subsystem5/1(EXT) -> TIM_Serv_Informatico_1 (344)/6  "EXT_SERVICE"
  [SERVIZI_ELE1] -> Subsystem5/1(servizio)
  [CYBER_RISK] -> TELCO1_org (542)/5  "CYBER_RISK"
  delay1/1(out) -> SERVIZI_TELCO1/1
  CYBER_RISK/1 -> [CYBER_RISK]
  MinMax6/1 -> Mux/2, Mux/1  "NODO_CYBER_QoS"
  MinMax5/1 -> Mux1/2, Mux1/1  "NODO_CYBER_QoS"
  MinMax1/1 -> Mux2/2, Mux2/1  "NODO_CYBER_QoS"
